simulink model "SS_1029"  (R2014a)
settings: Solver=FixedStepDiscrete  StartTime=0.0  StopTime=5  FixedStep=0.0005  RelTol=1e-3
values from neighbouring files (symbols this model uses):
  APS_High_null = ecucoder_cal(APS_High_null)    [SS.m]
  APS_High_x = ecucoder_cal(APS_High_x)    [SS.m]
  APS_High_y = ecucoder_cal(APS_High_y)    [SS.m]
  APS_Low_null = ecucoder_cal(APS_Low_null)    [SS.m]
  APS_low_x = ecucoder_cal(APS_low_x)    [SS.m]
  APS_low_y = ecucoder_cal(APS_low_y)    [SS.m]
  BrakeSignal_cal = ecucoder_cal(BrakeSignal_cal)    [SS.m]
  CustomReduceFactor_cal = ecucoder_cal(CustomReduceFactor_cal)    [SS.m]
  Differential_cal = ecucoder_cal(Differential_cal)    [SS.m]
  LowSOCWarning_cal = ecucoder_cal(LowSOCWarning_cal)    [SS.m]
  MotorTemperatureHigh_cal = ecucoder_cal(MotorTemperatureHigh_cal)    [SS.m]
  MotorTemperatureLow_cal = ecucoder_cal(MotorTemperatureLow_cal)    [SS.m]
  OilPressure_x = ecucoder_cal(OilPressure_x)    [SS.m]
  OilPressure_y = ecucoder_cal(OilPressure_y)    [SS.m]
  PowerBias_cal = ecucoder_cal(PowerBias_cal)    [SS.m]
  SpeedLimitFactor_x = ecucoder_cal(SpeedLimitFactor_x)    [SS.m]
  SpeedLimitFactor_y = ecucoder_cal(SpeedLimitFactor_y)    [SS.m]
  TorqueLimitNegativ_cal = ecucoder_cal(TorqueLimitNegativ_cal)    [SS.m]
  TorqueLimitPositiv_cal = ecucoder_cal(TorqueLimitPositiv_cal)    [SS.m]
libraries: simulink x101, ec55xxlib x31
(part 3 of 3)

== system SS_1029/VCU_MCU/Enabled Subsystem/Torquearrengement/Differential_ ==
  TIT2 : Inport
  T3T4 : Inport  Port=2
  CAN0333OK : Inport  Port=3
  Differential : Inport  Port=4
  Compare To Constant : simulink/Logic and Bit Operations/Compare To Constant  relop===  const=1  OutDataTypeStr=boolean
  Gain : Gain  Gain=0.5  OutDataTypeStr=single
  Gain1 : Gain  Gain=0.5  OutDataTypeStr=single
  Switch : Switch  Criteria=u2 > Threshold
  Unit Delay : UnitDelay  InitialCondition=Differential_cal  SampleTime=-1
  T1 : Outport
  T2 : Outport  Port=2
  T3 : Outport  Port=3
  T4 : Outport  Port=4
  "Differential " : Outport  Port=5
  wires:
  TIT2/1 -> Gain/1
  Gain/1 -> T2/1, T1/1
  T3T4/1 -> Gain1/1
  Gain1/1 -> T3/1, T4/1
  CAN0333OK/1 -> Compare To Constant/1
  Differential/1 -> Switch/1
  Switch/1 -> Unit Delay/1, [Differential]
  Unit Delay/1 -> Switch/3
  Compare To Constant/1 -> Switch/2
  [Differential] -> "Differential "/1

== system SS_1029/VCU_MCU/Enabled Subsystem/Torquearrengement/Power Cal1 ==
  aim_torque : Inport
  "rotate speed " : Inport  Port=2
  Gain : Gain  Gain=0.0098
  Gain1 : Gain  Gain=1/9549  ParamDataTypeStr=single
  Product : Product  OutDataTypeStr=single
  power : Outport
  wires:
  aim_torque/1 -> Gain/1
  Gain/1 -> Product/1
  "rotate speed "/1 -> Product/2
  Product/1 -> Gain1/1
  Gain1/1 -> power/1

== system SS_1029/VCU_MCU/Enabled Subsystem/Torquearrengement/Power Cal2 ==
  aim_torque : Inport
  "rotate speed " : Inport  Port=2
  Gain : Gain  Gain=0.0098
  Gain1 : Gain  Gain=1/9549  ParamDataTypeStr=single
  Product : Product  OutDataTypeStr=single
  power : Outport
  wires:
  aim_torque/1 -> Gain/1
  Gain/1 -> Product/1
  "rotate speed "/1 -> Product/2
  Product/1 -> Gain1/1
  Gain1/1 -> power/1

== system SS_1029/VCU_MCU/Enabled Subsystem/Torquearrengement/Power Cal3 ==
  aim_torque : Inport
  "rotate speed " : Inport  Port=2
  Gain : Gain  Gain=0.0098
  Gain1 : Gain  Gain=1/9549  ParamDataTypeStr=single
  Product : Product  OutDataTypeStr=single
  power : Outport
  wires:
  aim_torque/1 -> Gain/1
  Gain/1 -> Product/1
  "rotate speed "/1 -> Product/2
  Product/1 -> Gain1/1
  Gain1/1 -> power/1

== system SS_1029/VCU_MCU/Enabled Subsystem/Torquearrengement/Power Cal4 ==
  aim_torque : Inport
  "rotate speed " : Inport  Port=2
  Gain : Gain  Gain=0.0098
  Gain1 : Gain  Gain=1/9549  ParamDataTypeStr=single
  Product : Product  OutDataTypeStr=single
  power : Outport
  wires:
  aim_torque/1 -> Gain/1
  Gain/1 -> Product/1
  "rotate speed "/1 -> Product/2
  Product/1 -> Gain1/1
  Gain1/1 -> power/1

== system SS_1029/VCU_MCU/Enabled Subsystem/Torquearrengement/PowerBias_ ==
  TqSum : Inport
  PowerBias : Inport  Port=2
  CAN0333OK : Inport  Port=3
  Add : Sum  Inputs=+-
  Compare To Constant : simulink/Logic and Bit Operations/Compare To Constant  relop===  const=1  OutDataTypeStr=boolean
  Constant2 : Constant  OutDataTypeStr=single  SampleTime=-1
  Gain : Gain  Gain=80
  Product : Product
  Product1 : Product
  Saturation : Saturate  UpperLimit=1  LowerLimit=0  LinearizeAsGain=off
  Saturation1 : Saturate  UpperLimit=1  LowerLimit=0  LinearizeAsGain=off
  Switch : Switch  Criteria=u2 > Threshold
  Unit Delay : UnitDelay  InitialCondition=PowerBias_cal  SampleTime=-1
  T1T2 : Outport
  T3T4 : Outport  Port=2
  "PowerBias " : Outport  Port=3
  wires:
  TqSum/1 -> Gain/1
  Product/1 -> T1T2/1
  Product1/1 -> T3T4/1
  Add/1 -> Saturation1/1
  [PowerBias] -> Add/2
  Constant2/1 -> Add/1
  CAN0333OK/1 -> Compare To Constant/1
  PowerBias/1 -> Switch/1
  Switch/1 -> [PowerBias], Unit Delay/1
  Unit Delay/1 -> Switch/3
  Compare To Constant/1 -> Switch/2
  [PowerBias] -> "PowerBias "/1
  Gain/1 -> Product1/2, Product/2
  [PowerBias] -> Saturation/1
  Saturation/1 -> Product/1  "FrontPowerBias_mea"
  Saturation1/1 -> Product1/1  "RearPowerBias_mea"

== system SS_1029/HardWare_Input/In1_Message/Function-Call Subsystem/Subsystem1/Subsystem ==
  In1 : Inport
  Bitwise Operator : simulink/Logic and Bit Operations/Bitwise Operator  logicop=AND  UseBitMask=on  BitMask=bin2dec('00000001')  BitMaskRealWorld=Stored Integer
  Bitwise Operator1 : simulink/Logic and Bit Operations/Bitwise Operator  logicop=AND  UseBitMask=on  BitMask=bin2dec('00000010')  BitMaskRealWorld=Stored Integer
  Bitwise Operator2 : simulink/Logic and Bit Operations/Bitwise Operator  logicop=AND  UseBitMask=on  BitMask=bin2dec('00001000')  BitMaskRealWorld=Stored Integer
  Bitwise Operator3 : simulink/Logic and Bit Operations/Bitwise Operator  logicop=AND  UseBitMask=on  BitMask=bin2dec('00100000')  BitMaskRealWorld=Stored Integer
  Shift Arithmetic1 : ArithShift  BitShiftNumber=3  BitShiftDirection=Right
  Shift Arithmetic2 : ArithShift  BitShiftNumber=1  BitShiftDirection=Right
  Shift Arithmetic3 : ArithShift  BitShiftNumber=5  BitShiftDirection=Right
  AMK_bSystemReady : Outport
  AMK_bError : Outport  Port=2
  AMK_bQuitDcOn : Outport  Port=3
  AMK_bQuitInverterOn : Outport  Port=4
  wires:
  Bitwise Operator1/1 -> Shift Arithmetic2/1
  Bitwise Operator/1 -> AMK_bSystemReady/1
  In1/1 -> Bitwise Operator3/1, Bitwise Operator2/1, Bitwise Operator1/1, Bitwise Operator/1
  Shift Arithmetic2/1 -> AMK_bError/1
  Bitwise Operator2/1 -> Shift Arithmetic1/1
  Shift Arithmetic1/1 -> AMK_bQuitDcOn/1
  Bitwise Operator3/1 -> Shift Arithmetic3/1
  Shift Arithmetic3/1 -> AMK_bQuitInverterOn/1

== system SS_1029/HardWare_Input/In2_Message/Function-Call Subsystem/Subsystem1/Subsystem ==
  In1 : Inport
  Bitwise Operator : simulink/Logic and Bit Operations/Bitwise Operator  logicop=AND  UseBitMask=on  BitMask=bin2dec('00000001')  BitMaskRealWorld=Stored Integer
  Bitwise Operator1 : simulink/Logic and Bit Operations/Bitwise Operator  logicop=AND  UseBitMask=on  BitMask=bin2dec('00000010')  BitMaskRealWorld=Stored Integer
  Bitwise Operator2 : simulink/Logic and Bit Operations/Bitwise Operator  logicop=AND  UseBitMask=on  BitMask=bin2dec('00001000')  BitMaskRealWorld=Stored Integer
  Bitwise Operator3 : simulink/Logic and Bit Operations/Bitwise Operator  logicop=AND  UseBitMask=on  BitMask=bin2dec('00100000')  BitMaskRealWorld=Stored Integer
  Shift Arithmetic1 : ArithShift  BitShiftNumber=3  BitShiftDirection=Right
  Shift Arithmetic2 : ArithShift  BitShiftNumber=1  BitShiftDirection=Right
  Shift Arithmetic3 : ArithShift  BitShiftNumber=5  BitShiftDirection=Right
  AMK_bSystemReady : Outport
  AMK_bError : Outport  Port=2
  AMK_bQuitDcOn : Outport  Port=3
  AMK_bQuitInverterOn : Outport  Port=4
  wires:
  Bitwise Operator1/1 -> Shift Arithmetic2/1
  Bitwise Operator/1 -> AMK_bSystemReady/1
  In1/1 -> Bitwise Operator3/1, Bitwise Operator2/1, Bitwise Operator1/1, Bitwise Operator/1
  Shift Arithmetic2/1 -> AMK_bError/1
  Bitwise Operator2/1 -> Shift Arithmetic1/1
  Shift Arithmetic1/1 -> AMK_bQuitDcOn/1
  Bitwise Operator3/1 -> Shift Arithmetic3/1
  Shift Arithmetic3/1 -> AMK_bQuitInverterOn/1

== system SS_1029/HardWare_Input/In3_Message/Function-Call Subsystem/Subsystem1/Subsystem ==
  In1 : Inport
  Bitwise Operator : simulink/Logic and Bit Operations/Bitwise Operator  logicop=AND  UseBitMask=on  BitMask=bin2dec('00000001')  BitMaskRealWorld=Stored Integer
  Bitwise Operator1 : simulink/Logic and Bit Operations/Bitwise Operator  logicop=AND  UseBitMask=on  BitMask=bin2dec('00000010')  BitMaskRealWorld=Stored Integer
  Bitwise Operator2 : simulink/Logic and Bit Operations/Bitwise Operator  logicop=AND  UseBitMask=on  BitMask=bin2dec('00001000')  BitMaskRealWorld=Stored Integer
  Bitwise Operator3 : simulink/Logic and Bit Operations/Bitwise Operator  logicop=AND  UseBitMask=on  BitMask=bin2dec('00100000')  BitMaskRealWorld=Stored Integer
  Shift Arithmetic1 : ArithShift  BitShiftNumber=3  BitShiftDirection=Right
  Shift Arithmetic2 : ArithShift  BitShiftNumber=1  BitShiftDirection=Right
  Shift Arithmetic3 : ArithShift  BitShiftNumber=5  BitShiftDirection=Right
  AMK_bSystemReady : Outport
  AMK_bError : Outport  Port=2
  AMK_bQuitDcOn : Outport  Port=3
  AMK_bQuitInverterOn : Outport  Port=4
  wires:
  Bitwise Operator1/1 -> Shift Arithmetic2/1
  Bitwise Operator/1 -> AMK_bSystemReady/1
  In1/1 -> Bitwise Operator3/1, Bitwise Operator2/1, Bitwise Operator1/1, Bitwise Operator/1
  Shift Arithmetic2/1 -> AMK_bError/1
  Bitwise Operator2/1 -> Shift Arithmetic1/1
  Shift Arithmetic1/1 -> AMK_bQuitDcOn/1
  Bitwise Operator3/1 -> Shift Arithmetic3/1
  Shift Arithmetic3/1 -> AMK_bQuitInverterOn/1

== system SS_1029/HardWare_Input/In4_Message/Function-Call Subsystem/Subsystem1/Subsystem ==
  In1 : Inport
  Bitwise Operator : simulink/Logic and Bit Operations/Bitwise Operator  logicop=AND  UseBitMask=on  BitMask=bin2dec('00000001')  BitMaskRealWorld=Stored Integer
  Bitwise Operator1 : simulink/Logic and Bit Operations/Bitwise Operator  logicop=AND  UseBitMask=on  BitMask=bin2dec('00000010')  BitMaskRealWorld=Stored Integer
  Bitwise Operator2 : simulink/Logic and Bit Operations/Bitwise Operator  logicop=AND  UseBitMask=on  BitMask=bin2dec('00001000')  BitMaskRealWorld=Stored Integer
  Bitwise Operator3 : simulink/Logic and Bit Operations/Bitwise Operator  logicop=AND  UseBitMask=on  BitMask=bin2dec('00100000')  BitMaskRealWorld=Stored Integer
  Shift Arithmetic1 : ArithShift  BitShiftNumber=3  BitShiftDirection=Right
  Shift Arithmetic2 : ArithShift  BitShiftNumber=1  BitShiftDirection=Right
  Shift Arithmetic3 : ArithShift  BitShiftNumber=5  BitShiftDirection=Right
  AMK_bSystemReady : Outport
  AMK_bError : Outport  Port=2
  AMK_bQuitDcOn : Outport  Port=3
  AMK_bQuitInverterOn : Outport  Port=4
  wires:
  Bitwise Operator1/1 -> Shift Arithmetic2/1
  Bitwise Operator/1 -> AMK_bSystemReady/1
  In1/1 -> Bitwise Operator3/1, Bitwise Operator2/1, Bitwise Operator1/1, Bitwise Operator/1
  Shift Arithmetic2/1 -> AMK_bError/1
  Bitwise Operator2/1 -> Shift Arithmetic1/1
  Shift Arithmetic1/1 -> AMK_bQuitDcOn/1
  Bitwise Operator3/1 -> Shift Arithmetic3/1
  Shift Arithmetic3/1 -> AMK_bQuitInverterOn/1

== stateflow chart SS_1029/VCU_MCU/Enabled Subsystem/Chart1 ==
  state Normal
    entry:
    Logicvalue = single(1);
  state TimeCounting
    entry:
    Logicvalue = single(1);
  state Warning
    entry:
    Logicvalue = single(0);
  (default) -> Normal
  Warning -> Normal : [APPS_PCT<=5]
  Normal -> TimeCounting : [BrakeSignal==1&APPS_PCT>=15]
  TimeCounting -> Normal [order 1] : [BrakeSignal==0||APPS_PCT<15]
  TimeCounting -> Warning [order 2] : after(40,tick)
  data: BrakeSignal input; APPS_PCT input; Logicvalue output

== stateflow chart SS_1029/VCU_MCU/Enabled Subsystem/DRS Strategy ==
  state DRSOFF
    entry:
    DRSState=uint8(0);
  state DRSON
    entry:
    DRSState=uint8(1);
  (default) -> DRSOFF
  DRSOFF -> DRSON : [DRSCMD==1&&BrakeSignal==0]
  DRSON -> DRSOFF : [DRSCMD==0||BrakeSignal==1]
  data: BrakeSignal input; DRSCMD input; DRSState output

== stateflow chart SS_1029/VCU_MCU/Enabled Subsystem/Torquearrengement/Chart ==
  (default) -> (junction 6)
  (junction 6) -> (junction 5) [order 1] : [powersum<=53.3]
  (junction 6) -> (junction 7) [order 2] : {factor=single(53.3/powersum);}
  (junction 5) -> (junction 4) : {factor=single(1);}
  (junction 4) -> (junction 7)
  (junction 7) -> (junction 3)
  data: powersum input single; factor output single

== stateflow chart SS_1029/VCU_MCU/Enabled Subsystem/BuzzingLogic ==
  state Standby
    entry:
    AMK_InverterOn=uint8(1);
    AMK_DcOn= uint8(1);
    AMK_Enable= uint8(0);
    AMK_ErrorReset= uint8(0);
    AMK_TorqueLimitPositiv= int16(0);
    AMK_TorqueLimitNegativ= int16(0);
    Buzzing= uint8(0);
  state Running
    entry:
    AMK_InverterOn=uint8(1);
    AMK_DcOn= uint8(1);
    AMK_Enable= uint8(1);
    AMK_ErrorReset= uint8(0);
    AMK_TorqueLimitPositiv=int16(TorqueLimitPositiv_cal);
    AMK_TorqueLimitNegativ=int16(TorqueLimitNegativ_cal);
    Buzzing= uint8(0);
  state BrakeStandby
    entry:
    AMK_InverterOn=uint8(1);
    AMK_DcOn=uint8(1);
    AMK_Enable=uint8(0);
    AMK_ErrorReset=uint8(0);
    AMK_TorqueLimitPositiv=int16(0);
    AMK_TorqueLimitNegativ=int16(0);
    Buzzing=uint8(0);
  state MotorSpeedReq
    entry:
    AMK_InverterOn=uint8(1);
    AMK_DcOn=uint8(1);
    AMK_Enable=uint8(0);
    AMK_ErrorReset=uint8(0);
    AMK_TorqueLimitPositiv=int16(0);
    AMK_TorqueLimitNegativ=int16(0);
    Buzzing= uint8(0);
  state Buzzing
    entry:
    AMK_InverterOn=uint8(1);
    AMK_DcOn= uint8(1);
    AMK_Enable= uint8(1);
    AMK_ErrorReset= uint8(0);
    AMK_TorqueLimitPositiv= int16(0);
    AMK_TorqueLimitNegativ= int16(0);
    Buzzing= uint8(1);
  (default) -> Standby
  Running -> Standby : [StartSignal==0]
  Standby -> BrakeStandby : [BrakeSignal==1&StartSignal==0]
  BrakeStandby -> Standby [order 2] : [StartSignal==1&BrakeSignal==0]
  Buzzing -> Running : after(200,tick)
  BrakeStandby -> MotorSpeedReq [order 1] : [BrakeSignal==1&StartSignal==1]
  MotorSpeedReq -> Buzzing : after(100,tick)
  data: AMK_InverterOn output uint8; AMK_DcOn output uint8; AMK_Enable output uint8; AMK_ErrorReset output uint8; AMK_TorqueLimitPositiv output int16; AMK_TorqueLimitNegativ output int16; StartSignal input boolean; Buzzing output uint8; BrakeSignal input boolean; TorqueLimitPositiv_cal input; TorqueLimitNegativ_cal input
